simulink model "Problem3"  (R2020a)
settings: Solver=VariableStepAuto  StartTime=0.0  StopTime=100.0  RelTol=1e-3
settings Model: Creator=kasutav  LastModifiedBy=kasutav

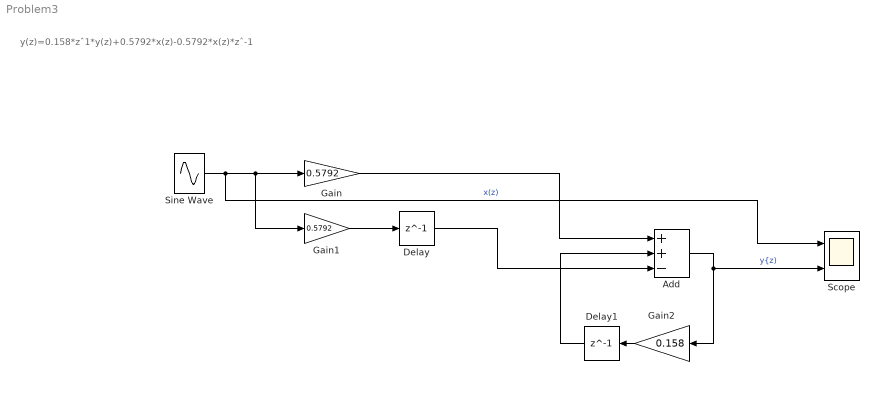
== system Problem3 ==
  note: y(z)=0.158*zˆ1*y(z)+0.5792*x(z)-0.5792*x(z)*zˆ-1
  Add : Sum  Inputs=++-
  Delay : Delay  DelayLength=1
  Delay1 : Delay  DelayLength=1
  Gain : Gain  Gain=0.5792
  Gain1 : Gain  Gain=0.5792
  Gain2 : Gain  Gain=0.158
  Scope : Scope  NumInputPorts=2
  Sine Wave : Sin  Frequency=62  SampleTime=0
  wires:
  Sine Wave/1 -> Scope/1, Gain1/1, Gain/1  "x(z)"
  Add/1 -> Scope/2, Gain2/1  "y{z)"
  Gain1/1 -> Delay/1
  Gain/1 -> Add/1
  Delay/1 -> Add/3
  Gain2/1 -> Delay1/1
  Delay1/1 -> Add/2
